simulink model "sampleModel1565"  (R2023a)
settings: Solver=VariableStepAuto  StartTime=0.0  StopTime=10.0  RelTol=1e-3
libraries: hdlsllib x3, simulink x1
settings Model: Creator=user1  LastModifiedBy=user1

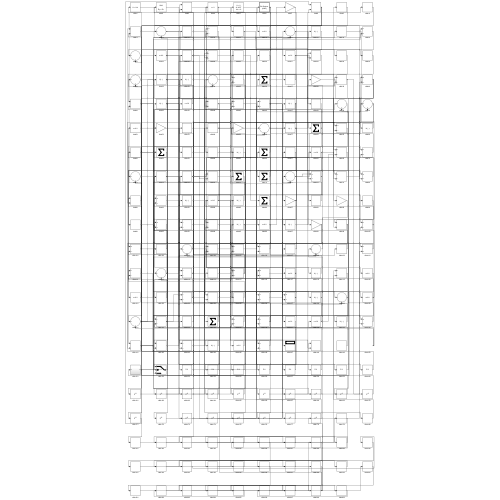
[thumbnail: Simulink's stored preview of the top-level diagram]
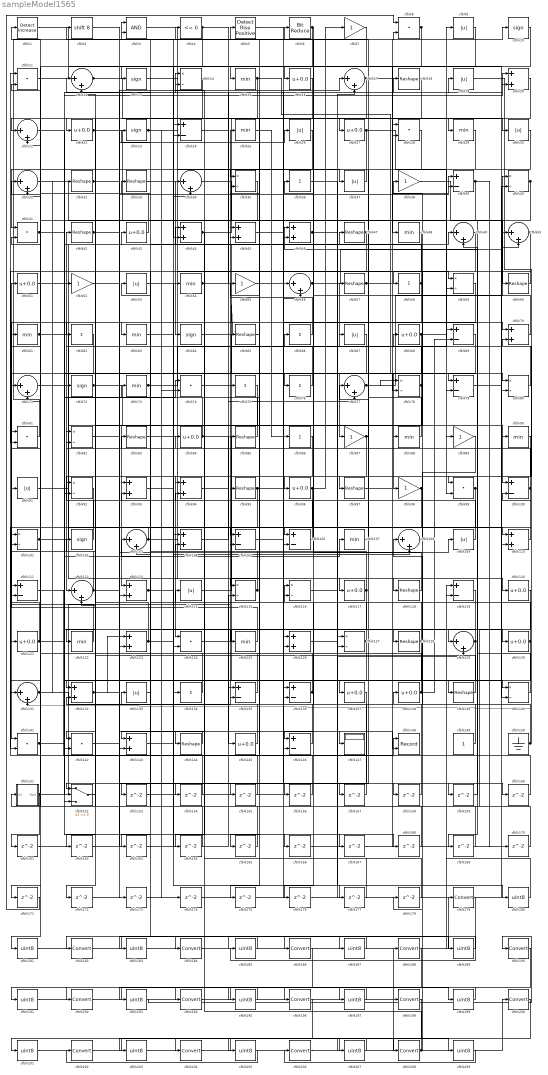
== system sampleModel1565 ==
  cfblk1 : simulink/Logic and Bit Operations/Detect Increase  vinit=0.0  OutDataTypeStr=boolean
      settings: LibrarySourceBlock=|
      | hdlsllib/Logic and Bit
      | Operations/Detect
      | Increase
  cfblk{10,13,23,64,72,102} (6 alike) : Signum
  cfblk{24,39,69,79,100,105..106,111,119,135..136,146} (12 alike) : Sum  Inputs=+-
  cfblk{14,35,40,59,78,80,82,92,101,115..116,127,140} (13 alike) : Product  Inputs=*/  RndMeth=Zero  SaturateOnIntegerOverflow=on
  cfblk{12,17,21,31,34,49..50,56,71,77,103,108,112,129,131} (15 alike) : Sum  Inputs=|++
  cfblk{20,44..46,70,93..94,104,110,113,123,126,132,143} (14 alike) : Sum
  cfblk{15,25,29,48,54,61,63,73,88,90,107,122,125} (13 alike) : MinMax
  cfblk{9,19,26,30,37,53,67,91,109,114,133} (11 alike) : Abs  SaturateOnIntegerOverflow=off
  cfblk{8,11,28,41,74,81,99,124,141..142} (10 alike) : DotProduct  OutDataTypeStr=Inherit: Inherit via internal rule
  cfblk{16,22,27,43,51,68,84,96,117,120..121,130,137..138,145} (15 alike) : Bias  Bias=0.0  SaturateOnIntegerOverflow=off
  cfblk{18,32..33,42,47,57,60,65,83,85,95,97,118,128,139,144} (16 alike) : Reshape
  cfblk{36,58,62,66,75..76,86,134} (8 alike) : Sum  Inputs=+
  cfblk147 : Display
  cfblk148 : Record  FileSettingsInternal="{\"entries\":[{\"content\":{\"excelSettings\":{\"content\":{},\"type\":\"Streamout.ExcelSettings\"}},\"type\":\"Streamout.FileSettingStorage\",\"uuid\":\"\"}],\"packageUris\":[\"http:\\/\\/schema.mathworks.com\\/mf0\\/streamout_blocks\\/R2020a\"],\"version\":\"1.0\"}"  Layout=[1 1]  SignalsInternal="{\"entries\":[{\"content\":{\"signals\":[{\"content\":{\"blockPath\":[],\"dimensions\":[1],\"domain\":\"\",\"lineColor\":\"#a2142f\",\"plots\":[1],\"port\":1,\"signalID\":1719,\"signalName\":\"XY Graph:1\"},\"type\":\"RecordBlkView.Signal\",\"uuid\":\"\"},{\"content\":{\"blockPath\":[],\"dimensions\":[1],\"domain\":\"\",\"lineColor\":\"#139fff\",\"plots\":[1],\"port\":2,\"signalID\":1722,\"signalName\":\"XY Graph:2\"},\"type\":\"RecordBlkView.Signal\",\"uuid\":\"\"}]},\"type\":\"RecordBlkView.InputSignals\",\"uuid\":\"\"}],\"packageUris\":[\"http:\\/\\/schema.mathworks.com\\/mf0\\/streamout_blocks\\/R2020a\"],\"version\":\"1.0\"}"  VisualizationBindings="{\"xyplotplugin\":{\"info\":[{\"series\":[{\"bindingParametersList\":[{\"parameter\":\"X-Axis\",\"signalID\":1719,\"signalName\":\"XY Graph:1\"},{\"parameter\":\"Y-Axis\",\"signalID\":1722,\"signalName\":\"XY Graph:2\"}],\"seriesID\":40114}],\"subplotID\":1}]}}"  CompatibilityTag=XY  st=-1
  cfblk149 : Constant  SampleTime=-1
  cfblk150 : Ground
  cfblk151 : Subsystem
      settings: LibrarySourceBlock=|
      | hdlsllib/Ports &
      | Subsystems/Subsystem
  cfblk152 : Switch  SaturateOnIntegerOverflow=off  InputSameDT=off
  cfblk{153..178} (26 alike) : Delay  SampleTime=1
  cfblk{179,182,184,186,188,190,192,194,196,198,200,202,204,206,208} (15 alike) : DataTypeConversion  SaturateOnIntegerOverflow=off  RndMeth=Floor
  cfblk{180..181,183,185,187,189,191,193,195,197,199,201,203,205,207,209} (16 alike) : DataTypeConversion  OutDataTypeStr=uint8  SaturateOnIntegerOverflow=off  RndMeth=Floor
  cfblk2 : ArithShift  BitShiftNumber=8
  cfblk3 : Logic  AllPortsSameDT=off  OutDataTypeStr=boolean
  cfblk{7,38,52,55,87,89,98} (7 alike) : Gain
  cfblk4 : hdlsllib/Logic and Bit Operations/Compare To Zero  relop=<=  OutDataTypeStr=boolean
  cfblk5 : hdlsllib/Logic and Bit Operations/Detect Rise Positive  vinit=0  OutDataTypeStr=boolean
  cfblk6 : hdlsllib/Logic and Bit Operations/Bit Reduce  mode=AND
  wires:
  cfblk87/1 -> cfblk112/1, cfblk67/1
  cfblk25/1 -> cfblk86/1
  cfblk60/1 -> cfblk58/1
  cfblk44/1 -> cfblk27/1, cfblk144/1
  cfblk11/1 -> cfblk16/1
  cfblk15/1 -> cfblk79/1, cfblk44/2
  cfblk81/1 -> cfblk6/1
  cfblk144/1 -> cfblk143/1
  cfblk51/1 -> cfblk49/1
  cfblk75/1 -> cfblk113/1
  cfblk121/1 -> cfblk51/1, cfblk74/1
  cfblk101/1 -> cfblk43/1, cfblk61/1
  cfblk86/1 -> cfblk124/1
  cfblk13/1 -> cfblk117/1
  cfblk53/1 -> cfblk134/1
  cfblk19/1 -> cfblk99/1
  cfblk71/1 -> cfblk143/2
  cfblk14/1 -> cfblk21/1
  cfblk127/1 -> cfblk104/2, cfblk153/1
  cfblk111/1 -> cfblk148/1
  cfblk83/1 -> cfblk118/1
  cfblk89/1 -> cfblk133/1
  cfblk114/1 -> cfblk66/1
  cfblk6/1 -> cfblk96/1, cfblk71/2
  cfblk66/1 -> cfblk25/1
  cfblk28/1 -> cfblk41/1
  cfblk124/1 -> cfblk129/1
  cfblk33/1 -> cfblk64/1
  cfblk90/1 -> cfblk94/1
  cfblk67/1 -> cfblk146/1
  cfblk133/1 -> cfblk53/1
  cfblk59/1 -> cfblk141/1
  cfblk109/1 -> cfblk42/1
  cfblk96/1 -> cfblk7/1, cfblk164/1
  cfblk55/1 -> cfblk18/1
  cfblk77/1 -> cfblk40/1, cfblk78/1
  cfblk102/1 -> cfblk82/1
  cfblk74/1 -> cfblk47/1
  cfblk73/1 -> cfblk9/1, cfblk46/2, cfblk174/1
  cfblk61/1 -> cfblk100/1, cfblk123/2
  cfblk8/1 -> cfblk76/1, cfblk28/2, cfblk21/2
  cfblk143/1 -> cfblk54/1
  cfblk92/1 -> cfblk141/2
  cfblk62/1 -> cfblk121/1
  cfblk22/1 -> cfblk126/1, cfblk130/1
  cfblk95/1 -> cfblk152/2, cfblk159/1
  cfblk85/1 -> cfblk33/1
  cfblk84/1 -> cfblk136/2, cfblk147/1, cfblk3/2
  cfblk37/1 -> cfblk35/1
  cfblk3/1 -> cfblk89/1
  cfblk17/1 -> cfblk29/1, cfblk131/1
  cfblk115/1 -> cfblk12/1, cfblk72/1
  cfblk5/1 -> cfblk70/1
  cfblk151/1(Out1) -> cfblk45/1, cfblk14/2, cfblk161/1
  cfblk135/1 -> cfblk114/1
  cfblk100/1 -> cfblk139/1, cfblk12/2
  cfblk120/1 -> cfblk151/1(In1)
  cfblk145/1 -> cfblk95/1
  cfblk110/1 -> cfblk105/1
  cfblk9/1 -> cfblk15/1
  cfblk47/1 -> cfblk63/1, cfblk81/2
  cfblk79/1 -> cfblk40/2
  cfblk103/1 -> cfblk101/1, cfblk116/2
  cfblk18/1 -> cfblk22/1
  cfblk142/1 -> cfblk26/1
  cfblk128/1 -> cfblk23/1, cfblk142/2
  cfblk68/1 -> cfblk87/1, cfblk80/1
  cfblk94/1 -> cfblk110/1
  cfblk132/1 -> cfblk39/1, cfblk123/1
  cfblk58/1 -> cfblk3/1, cfblk171/1
  cfblk1/1 -> cfblk90/1
  cfblk104/1 -> cfblk85/1
  cfblk152/1 -> cfblk82/2
  cfblk43/1 -> cfblk11/2
  cfblk69/1 -> cfblk91/1
  cfblk78/1 -> cfblk35/2, cfblk172/1
  cfblk52/1 -> cfblk148/2
  cfblk21/1 -> cfblk137/1
  cfblk113/1 -> cfblk8/2, cfblk73/1
  cfblk117/1 -> cfblk75/1, cfblk175/1
  cfblk122/1 -> cfblk111/1
  cfblk39/1 -> cfblk79/2, cfblk170/1
  cfblk64/1 -> cfblk98/1
  cfblk57/1 -> cfblk10/1, cfblk97/1
  cfblk20/1 -> cfblk115/1
  cfblk38/1 -> cfblk60/1
  cfblk31/1 -> cfblk69/1
  cfblk108/1 -> cfblk38/1
  cfblk98/1 -> cfblk106/1, cfblk154/1
  cfblk27/1 -> cfblk48/1, cfblk59/2, cfblk92/2
  cfblk54/1 -> cfblk65/1, cfblk19/1
  cfblk118/1 -> cfblk36/1
  cfblk129/1 -> cfblk125/1, cfblk152/3
  cfblk76/1 -> cfblk52/1
  cfblk149/1 -> cfblk116/1
  cfblk70/1 -> cfblk2/1
  cfblk140/1 -> cfblk46/1
  cfblk40/1 -> cfblk71/1, cfblk140/2, cfblk169/1
  cfblk150/1 -> cfblk100/2, cfblk138/1, cfblk131/2
  cfblk97/1 -> cfblk39/2
  cfblk63/1 -> cfblk34/1
  cfblk139/1 -> cfblk102/1
  cfblk146/1 -> cfblk5/1
  cfblk49/1 -> cfblk88/1
  cfblk141/1 -> cfblk45/2, cfblk166/1, cfblk167/1
  cfblk12/1 -> cfblk145/1, cfblk120/1
  cfblk134/1 -> cfblk83/1
  cfblk88/1 -> cfblk4/1
  cfblk56/1 -> cfblk50/1, cfblk129/2
  cfblk16/1 -> cfblk62/1
  cfblk48/1 -> cfblk146/2
  cfblk10/1 -> cfblk13/1
  cfblk42/1 -> cfblk142/1, cfblk124/2, cfblk17/1
  cfblk130/1 -> cfblk70/2, cfblk44/1, cfblk176/1
  cfblk138/1 -> cfblk14/1, cfblk69/2
  cfblk23/1 -> cfblk37/1, cfblk74/2
  cfblk136/1 -> cfblk31/1, cfblk93/2
  cfblk4/1 -> cfblk77/2, cfblk181/1
  cfblk99/1 -> cfblk122/1, cfblk163/1
  cfblk105/1 -> cfblk56/2
  cfblk34/1 -> cfblk99/2
  cfblk80/1 -> cfblk57/1
  cfblk7/1 -> cfblk24/2
  cfblk30/1 -> cfblk132/1
  cfblk32/1 -> cfblk80/2, cfblk158/1
  cfblk72/1 -> cfblk135/1, cfblk128/1
  cfblk123/1 -> cfblk92/1, cfblk108/2
  cfblk41/1 -> cfblk20/1, cfblk78/2
  cfblk107/1 -> cfblk77/1
  cfblk137/1 -> cfblk152/1
  cfblk36/1 -> cfblk140/1
  cfblk106/1 -> cfblk55/1
  cfblk126/1 -> cfblk68/1
  cfblk131/1 -> cfblk135/2, cfblk32/1, cfblk107/1, cfblk20/2
  cfblk91/1 -> cfblk127/2
  cfblk24/1 -> cfblk30/1
  cfblk125/1 -> cfblk111/2
  cfblk112/1 -> cfblk109/1, cfblk81/1
  cfblk50/1 -> cfblk103/2, cfblk93/1
  cfblk46/1 -> cfblk59/1, cfblk168/1
  cfblk153/1 -> cfblk56/1
  cfblk154/1 -> cfblk1/1
  cfblk26/1 -> cfblk155/1
  cfblk155/1 -> cfblk31/2
  cfblk82/1 -> cfblk156/1
  cfblk156/1 -> cfblk11/1
  cfblk29/1 -> cfblk157/1
  cfblk157/1 -> cfblk104/1
  cfblk158/1 -> cfblk112/2
  cfblk159/1 -> cfblk49/2
  cfblk45/1 -> cfblk160/1
  cfblk160/1 -> cfblk105/2
  cfblk161/1 -> cfblk115/2
  cfblk35/1 -> cfblk162/1
  cfblk162/1 -> cfblk113/2
  cfblk163/1 -> cfblk34/2
  cfblk164/1 -> cfblk103/1
  cfblk65/1 -> cfblk165/1
  cfblk165/1 -> cfblk24/1
  cfblk166/1 -> cfblk28/1
  cfblk167/1 -> cfblk110/2
  cfblk168/1 -> cfblk41/2
  cfblk169/1 -> cfblk132/2
  cfblk170/1 -> cfblk101/2
  cfblk171/1 -> cfblk8/1
  cfblk172/1 -> cfblk126/2
  cfblk2/1 -> cfblk173/1
  cfblk173/1 -> cfblk127/1
  cfblk174/1 -> cfblk17/2
  cfblk175/1 -> cfblk106/2
  cfblk176/1 -> cfblk50/2
  cfblk93/1 -> cfblk177/1
  cfblk177/1 -> cfblk136/1
  cfblk178/1 -> cfblk94/2
  cfblk116/1 -> cfblk180/1
  cfblk180/1 -> cfblk119/1
  cfblk181/1 -> cfblk119/2
  cfblk119/1 -> cfblk183/1
  cfblk183/1 -> cfblk179/1
  cfblk179/1 -> cfblk185/1
  cfblk185/1 -> cfblk182/1
  cfblk182/1 -> cfblk187/1
  cfblk187/1 -> cfblk184/1
  cfblk184/1 -> cfblk189/1
  cfblk189/1 -> cfblk186/1
  cfblk186/1 -> cfblk191/1
  cfblk191/1 -> cfblk188/1
  cfblk188/1 -> cfblk193/1
  cfblk193/1 -> cfblk190/1
  cfblk190/1 -> cfblk195/1
  cfblk195/1 -> cfblk192/1
  cfblk192/1 -> cfblk197/1
  cfblk197/1 -> cfblk194/1
  cfblk194/1 -> cfblk199/1
  cfblk199/1 -> cfblk196/1
  cfblk196/1 -> cfblk201/1
  cfblk201/1 -> cfblk198/1
  cfblk198/1 -> cfblk203/1
  cfblk203/1 -> cfblk200/1
  cfblk200/1 -> cfblk205/1
  cfblk205/1 -> cfblk202/1
  cfblk206/1 -> cfblk208/1
  cfblk202/1 -> cfblk207/1
  cfblk207/1 -> cfblk204/1
  cfblk208/1 -> cfblk178/1, cfblk108/1, cfblk84/1
  cfblk204/1 -> cfblk209/1
  cfblk209/1 -> cfblk206/1

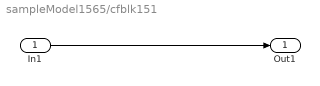
== system sampleModel1565/cfblk151 ==
  In1 : Inport
  Out1 : Outport
  wires:
  In1/1 -> Out1/1
